simulink model "seminar3questions"  (R2016a)
settings: Solver=VariableStepAuto  StartTime=0.0  StopTime=0.1  RelTol=1e-3
libraries: powerlib x17, powerlib_meascontrol x7
settings Model: Creator=lll  LastModifiedBy=lll

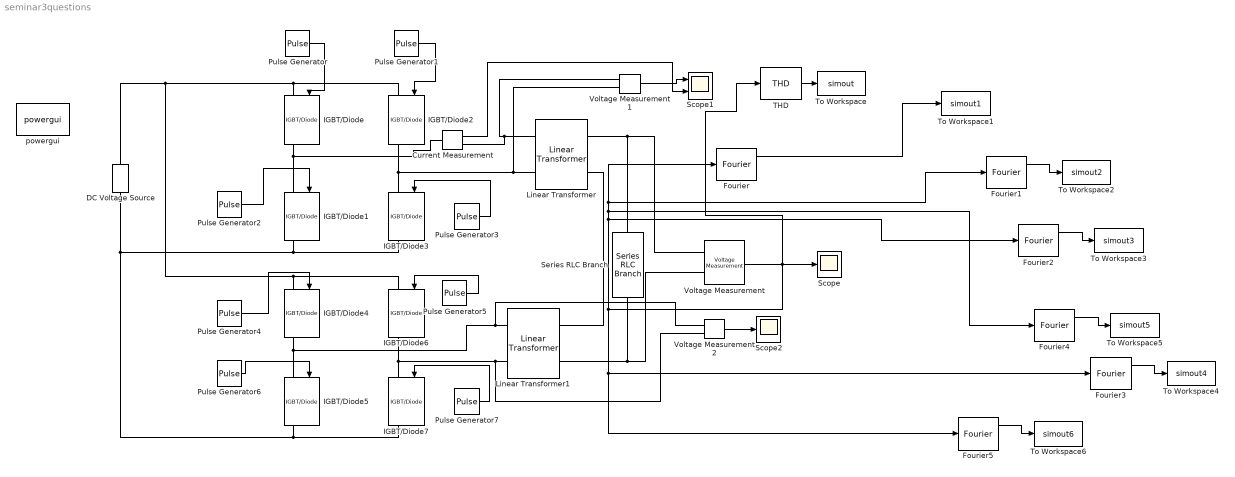
== system seminar3questions ==
  Current Measurement : powerlib/Measurements/Current Measurement  PhasorSimulation=off  OutputType=Complex  PSBequivalent=0
  DC Voltage Source : powerlib/Electrical Sources/DC Voltage Source  Amplitude=400  Measurements=None
  Fourier : powerlib_meascontrol/Measurements/Fourier  Freq=50  n=1  InInit=[0, 0]  Ts=0
  Fourier1 : powerlib_meascontrol/Measurements/Fourier  Freq=50  n=3  InInit=[0, 0]  Ts=0
  Fourier2 : powerlib_meascontrol/Measurements/Fourier  Freq=50  n=5  InInit=[0, 0]  Ts=0
  Fourier3 : powerlib_meascontrol/Measurements/Fourier  Freq=50  n=7  InInit=[0, 0]  Ts=0
  Fourier4 : powerlib_meascontrol/Measurements/Fourier  Freq=50  n=6  InInit=[0, 0]  Ts=0
  Fourier5 : powerlib_meascontrol/Measurements/Fourier  Freq=50  n=9  InInit=[0, 0]  Ts=0
  IGBT/Diode{,1..7} (8 alike) : powerlib/Power Electronics/IGBT//Diode  Ron=1e-3  Rs=1e5  Cs=inf  Measurements=on
  Linear Transformer : powerlib/Elements/Linear Transformer  UNITS=pu  NominalPower=[ 1e4 50 ]  winding1="[ 100  0.002  0.05 ]"  winding2="[ 100  0.002  0.05]"  ThreeWindings=off  winding3=[ 315e3 0.002 0.08 ]  RmLm=[ 500 500 ]  Measurements=None  DataType=off
  Linear Transformer1 : powerlib/Elements/Linear Transformer  UNITS=pu  NominalPower=[ 1e4 50 ]  winding1=[100 0.002 0.05]  winding2=[100 0.002 0.05]  ThreeWindings=off  winding3=[3.15e+05 0.002 0.066667]  RmLm=[500 500]  Measurements=None  DataType=off
  Pulse Generator : DiscretePulseGenerator  PulseType=Time based  Period=0.02  PulseWidth=50
  Pulse Generator1 : DiscretePulseGenerator  PulseType=Time based  Period=0.02  PulseWidth=50  PhaseDelay=0.008333
  Pulse Generator2 : DiscretePulseGenerator  PulseType=Time based  Period=0.02  PulseWidth=50  PhaseDelay=0.01
  Pulse Generator3 : DiscretePulseGenerator  PulseType=Time based  Period=0.02  PulseWidth=50  PhaseDelay=0.018333
  Pulse Generator4 : DiscretePulseGenerator  PulseType=Time based  Period=0.02  PulseWidth=50  PhaseDelay=0.003333
  Pulse Generator5 : DiscretePulseGenerator  PulseType=Time based  Period=0.02  PulseWidth=50  PhaseDelay=0.0116666
  Pulse Generator6 : DiscretePulseGenerator  PulseType=Time based  Period=0.02  PulseWidth=50  PhaseDelay=0.013333
  Pulse Generator7 : DiscretePulseGenerator  PulseType=Time based  Period=0.02  PulseWidth=50  PhaseDelay=0.021666
  Scope : Scope
  Scope1 : Scope  NumInputPorts=2
  Scope2 : Scope
  Series RLC Branch : powerlib/Elements/Series RLC Branch  LConnTagsString=__new0  RConnTagsString=__new0  BranchType=R  Resistance=8  Inductance=0  SetiL0=off  InitialCurrent=0  Capacitance=0  Setx0=off  InitialVoltage=0  Measurements=None
  THD : powerlib_meascontrol/Measurements/THD  Freq=50  Ts=0
  To Workspace : ToWorkspace  VariableName=simout  SaveFormat=Timeseries  SampleTime=-1
  To Workspace1 : ToWorkspace  VariableName=simout1  SaveFormat=Timeseries  SampleTime=-1
  To Workspace2 : ToWorkspace  VariableName=simout2  SaveFormat=Timeseries  SampleTime=-1
  To Workspace3 : ToWorkspace  VariableName=simout3  SaveFormat=Timeseries  SampleTime=-1
  To Workspace4 : ToWorkspace  VariableName=simout4  SaveFormat=Timeseries  SampleTime=-1
  To Workspace5 : ToWorkspace  VariableName=simout5  SaveFormat=Timeseries  SampleTime=-1
  To Workspace6 : ToWorkspace  VariableName=simout6  SaveFormat=Timeseries  SampleTime=-1
  Voltage Measurement : powerlib/Measurements/Voltage Measurement  PhasorSimulation=off  OutputType=Complex  PSBequivalent=0
  Voltage Measurement1 : powerlib/Measurements/Voltage Measurement  PhasorSimulation=off  OutputType=Complex  PSBequivalent=0
  Voltage Measurement2 : powerlib/Measurements/Voltage Measurement  PhasorSimulation=off  OutputType=Complex  PSBequivalent=0
  powergui : powerlib/powergui  Priority=1  SimulationMode=Continuous  SolverType=Tustin/Backward Euler (TBE)  SampleTime=50e-6  frequency=60  SPID=off  DisableSnubberDevices=off  DisableRonSwitches=off  DisableVfSwitches=off  SwTol=0  DisplayEquations=off  Interpol=off  ExternalGateDelay=off  methode=off  Ts=10  FunctionMessages=off  echomessages=off  HookPort=off  EnableUseOfTLC=off  x0status=blocks  frequencyindice=0  Pbase=100e6  ErrMax=1e-4  Iterations=50  UnitsV=kV  UnitsW=MW  buscounter=0  RestoreLinks=warning  ResistiveCurrentMeasurement=off  Frange=[0:2:500]  Ylog=off  Xlog=on  ShowGrid=off  save=off  variable=ZData  structure=ScopeData  ZoomFFT=off  StartTime=0.0  cycles=1  DisplayStyle=1  fundamental=50  FreqAxis=off  MaxFrequency=1000  frequencyindicesteady=1  RmsSteady=1  display=off
  wires:
  Pulse Generator2/1 -> IGBT/Diode1/1
  Pulse Generator4/1 -> IGBT/Diode4/1
  Pulse Generator6/1 -> IGBT/Diode5/1
  Pulse Generator/1 -> IGBT/Diode/1
  Voltage Measurement1/1 -> Scope1/1
  Voltage Measurement2/1 -> Scope2/1
  Pulse Generator3/1 -> IGBT/Diode3/1
  Pulse Generator7/1 -> IGBT/Diode7/1
  Pulse Generator5/1 -> IGBT/Diode6/1
  Pulse Generator1/1 -> IGBT/Diode2/1
  Fourier/1 -> To Workspace1/1
  THD/1 -> To Workspace/1
  Current Measurement/1 -> Scope1/2
  Fourier1/1 -> To Workspace2/1
  Fourier2/1 -> To Workspace3/1
  Fourier3/1 -> To Workspace4/1
  Voltage Measurement/1 -> THD/1, Fourier3/1, Fourier5/1, Fourier/1, Fourier1/1, Fourier4/1, Fourier2/1, Scope/1
  Fourier4/1 -> To Workspace5/1
  Fourier5/1 -> To Workspace6/1
  connections:
  IGBT/Diode/RConn1 -- IGBT/Diode1/LConn1 -- Current Measurement/LConn1
  IGBT/Diode2/RConn1 -- Voltage Measurement1/LConn2 -- Linear Transformer/LConn2 -- IGBT/Diode3/LConn1
  IGBT/Diode/LConn1 -- IGBT/Diode6/LConn1 -- IGBT/Diode4/LConn1 -- DC Voltage Source/RConn1 -- IGBT/Diode2/LConn1
  IGBT/Diode3/RConn1 -- IGBT/Diode7/RConn1 -- IGBT/Diode5/RConn1 -- DC Voltage Source/LConn1 -- IGBT/Diode1/RConn1
  IGBT/Diode6/RConn1 -- Voltage Measurement2/LConn2 -- Linear Transformer1/LConn2 -- IGBT/Diode7/LConn1
  IGBT/Diode4/RConn1 -- Voltage Measurement2/LConn1 -- Linear Transformer1/LConn1 -- IGBT/Diode5/LConn1
  Linear Transformer/RConn2 -- Linear Transformer1/RConn1
  Linear Transformer/RConn1 -- Series RLC Branch/RConn1 -- Voltage Measurement/LConn1
  Voltage Measurement/LConn2 -- Series RLC Branch/LConn1 -- Linear Transformer1/RConn2
  Linear Transformer/LConn1 -- Current Measurement/RConn1 -- Voltage Measurement1/LConn1
